simulink model "model_hor_lin"  (R2020b)
settings: Solver=ode45  StartTime=0.0  StopTime=10  MaxStep=0.01  RelTol=1e-3
undefined symbols (not defined in the file): params
settings Model: Creator=Danil  LastModifiedBy=Danil

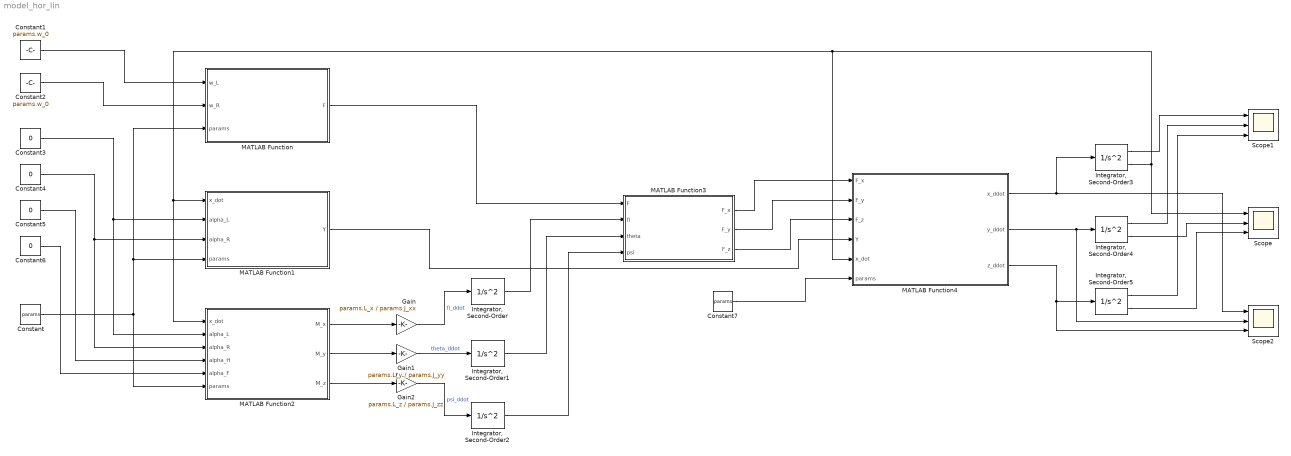
== system model_hor_lin ==
  Constant : Constant  Value=params  OutDataTypeStr=Bus: params_bus
  Constant1 : Constant  Value=params.w_0
  Constant2 : Constant  Value=params.w_0
  Constant{3..6} (4 alike) : Constant  Value=0
  Constant7 : Constant  Value=params  OutDataTypeStr=Bus: params_bus
  Gain : Gain  Gain=params.L_x / params.J_xx
  Gain1 : Gain  Gain=params.L_y / params.J_yy
  Gain2 : Gain  Gain=params.L_z / params.J_zz
  "Integrator, Second-Order" : SecondOrderIntegrator  ShowOutput=x
  "Integrator, Second-Order1" : SecondOrderIntegrator  ShowOutput=x
  "Integrator, Second-Order2" : SecondOrderIntegrator  ShowOutput=x
  "Integrator, Second-Order3" : SecondOrderIntegrator
  "Integrator, Second-Order4" : SecondOrderIntegrator
  "Integrator, Second-Order5" : SecondOrderIntegrator
  MATLAB Function : MATLAB Function  TreatAsAtomicUnit=on
  MATLAB Function1 : MATLAB Function  TreatAsAtomicUnit=on
  MATLAB Function2 : MATLAB Function  TreatAsAtomicUnit=on
  MATLAB Function3 : MATLAB Function  TreatAsAtomicUnit=on
  MATLAB Function4 : MATLAB Function  TreatAsAtomicUnit=on
  Scope : Scope  NumInputPorts=3
  Scope1 : Scope  NumInputPorts=3
  Scope2 : Scope  NumInputPorts=3
  wires:
  Constant/1 -> MATLAB Function/3(params), MATLAB Function1/4(params), MATLAB Function2/6(params)
  MATLAB Function2/1(M_x) -> Gain/1
  MATLAB Function2/2(M_y) -> Gain1/1
  MATLAB Function2/3(M_z) -> Gain2/1
  Gain/1 -> "Integrator, Second-Order"/1  "fi_ddot"
  Gain1/1 -> "Integrator, Second-Order1"/1  "theta_ddot"
  Gain2/1 -> "Integrator, Second-Order2"/1  "psi_ddot"
  MATLAB Function/1(F) -> MATLAB Function3/1(F)
  "Integrator, Second-Order"/1 -> MATLAB Function3/2(fi)
  "Integrator, Second-Order1"/1 -> MATLAB Function3/3(theta)
  "Integrator, Second-Order2"/1 -> MATLAB Function3/4(psi)
  MATLAB Function4/1(x_ddot) -> "Integrator, Second-Order3"/1, Scope2/1
  MATLAB Function4/2(y_ddot) -> Scope2/2, "Integrator, Second-Order4"/1
  MATLAB Function4/3(z_ddot) -> Scope2/3, "Integrator, Second-Order5"/1
  Constant1/1 -> MATLAB Function/1(w_L)
  Constant2/1 -> MATLAB Function/2(w_R)
  Constant3/1 -> MATLAB Function2/2(alpha_L), MATLAB Function1/2(alpha_L)
  Constant4/1 -> MATLAB Function2/3(alpha_R), MATLAB Function1/3(alpha_R)
  Constant5/1 -> MATLAB Function2/4(alpha_H)
  Constant6/1 -> MATLAB Function2/5(alpha_F)
  "Integrator, Second-Order3"/2 -> Scope/1, MATLAB Function4/5(x_dot), MATLAB Function2/1(x_dot), MATLAB Function1/1(x_dot)
  MATLAB Function3/1(F_x) -> MATLAB Function4/1(F_x)
  MATLAB Function3/2(F_y) -> MATLAB Function4/2(F_y)
  MATLAB Function3/3(F_z) -> MATLAB Function4/3(F_z)
  MATLAB Function1/1(Y) -> MATLAB Function4/4(Y)
  Constant7/1 -> MATLAB Function4/6(params)
  "Integrator, Second-Order3"/1 -> Scope1/1
  "Integrator, Second-Order4"/1 -> Scope1/2
  "Integrator, Second-Order5"/1 -> Scope1/3
  "Integrator, Second-Order4"/2 -> Scope/2
  "Integrator, Second-Order5"/2 -> Scope/3

== matlab function model_hor_lin/MATLAB Function1 ==
  data: x_dot input; alpha_L input; alpha_R input; params input; Y output
function Y = fcn(x_dot, alpha_L, alpha_R, params)

C_y_L = 0.1029 + 0.1498 * (alpha_L + 6.3236);
C_y_R = 0.1029 + 0.1498 * (alpha_R + 6.3236);
v = 196.4002 + 28.0286 * (x_dot - 14.0143);

Y = (1 / 2) * params.rho * v * params.S_k * (C_y_L + C_y_R);

== matlab function model_hor_lin/MATLAB Function ==
  data: w_L input; F output; w_R input; params input
function F  = fcn(w_L, w_R, params)
F = params.k_F * (w_L^2 + w_R^2);

== matlab function model_hor_lin/MATLAB Function2 ==
  data: x_dot input; M_x output; alpha_L input; alpha_R input; alpha_H input; alpha_F input; M_y output; M_z output; params input
function [M_x, M_y, M_z] = fcn(x_dot, alpha_L, alpha_R, alpha_H, alpha_F, params)

C_y_L = 0.1029 + 0.1498 * (alpha_L + 6.3236);
C_y_R = 0.1029 + 0.1498 * (alpha_R + 6.3236);
C_y_H = 0.12 * alpha_H;
C_y_F = 0.12 * alpha_F;
v = 196.4002 + 28.0286 * (x_dot - 14.0143);


M_x = (1 / 2) * params.rho * v * params.S_k * (C_y_L - C_y_R);
M_y = C_y_H * (1 / 2) * params.rho * v * params.S_h;
M_z = C_y_F * (1 / 2) * params.rho * v * params.S_f;

== matlab function model_hor_lin/MATLAB Function3 ==
  data: F input; F_x output; fi input; theta input; psi input; F_y output; F_z output
function [F_x, F_y, F_z] = fcn(F, fi, theta, psi)

F_x = F;
F_y = F * (cos(fi) * psi + sin(fi) * theta);
F_z = F * (sin(fi) * psi - cos(fi) * theta);

== matlab function model_hor_lin/MATLAB Function4 ==
  data: F_x input; x_ddot output; F_y input; F_z input; Y input; x_dot input; params input; y_ddot output; z_ddot output
function [x_ddot, y_ddot, z_ddot] = fcn(F_x, F_y, F_z, Y, x_dot, params)

x_ddot = (1 / params.m) * (F_x - params.k_x * x_dot);
y_ddot = (1 / params.m) * F_y;
z_ddot = (1 / params.m) * (F_z + Y - params.m * params.g);
